simulink model "SIL_Simulation_Parallel_Implementation"  (R2018b)
settings: Solver=FixedStepAuto  StartTime=0.0  StopTime=5  FixedStep=sim_step  RelTol=1e-3
values from neighbouring files (symbols this model uses):
  sim_step = 0.02    [main.m]
settings Model: ExtModeTrigDuration=200  Creator=young  LastModifiedBy=computation
settings DataIOCC: SaveOutput=off  SaveTime=off
settings OptimizationCC: DefaultParameterBehavior=Inlined  UseDivisionForNetSlopeComputation=on  UseFloatMulNetSlope=on  InlineInvariantSignals=on  EnhancedBackFolding=on  BooleansAsBitfields=on  PassReuseOutputArgsAs=Individual arguments  StateBitsets=on  DataBitsets=on  ZeroExternalMemoryAtStartup=off  ZeroInternalMemoryAtStartup=off  NoFixptDivByZeroProtection=on  EfficientFloat2IntCast=on  LifeSpan=1  OptimizeBlockOrder=speed  DifferentSizesBufferReuse=on
settings DebuggingCC: ParameterTunabilityLossMsg=error
settings HardwareCC: ProdBitPerPointer=32  ProdBitPerSizeT=32  ProdBitPerPtrDiffT=32  ProdLargestAtomicInteger=Integer  ProdWordSize=32  ProdLongLongMode=on  ProdHWDeviceType=Custom Processor
settings SFSimCC: SimUseLocalCustomCode=off  MATLABDynamicMemAlloc=off
settings RTWCC: SystemTargetFile=CompSOC_ec.tlc  TemplateMakefile=CompSOC_ec.tmf  Description=CompSOC EC Target  GenerateReport=on  RTWUseLocalCustomCode=off  IncludeHyperlinkInReport=on  LaunchReport=on  CreateSILPILBlock=PIL  CodeExecutionProfiling=on  CodeProfilingSaveOptions=AllData  CodeProfilingInstrumentation=detailed  GenerateTraceInfo=on  GenerateTraceReport=on  GenerateTraceReportSl=on  GenerateTraceReportSf=on  GenerateTraceReportEml=on  GenerateWebview=on  GenerateCodeMetricsReport=on
settings CodeAppCC: ForceParamTrailComments=on  IgnoreCustomStorageClasses=off  OperatorAnnotations=on  SimulinkDataObjDesc=on  SFDataObjDesc=on  CustomSymbolStrGlobalVar=rt$N$M  CustomSymbolStrType=$N$M  CustomSymbolStrFcn=$N$M$F  CustomSymbolStrMacro=$N$M  InsertBlockDesc=on
settings STFCustomTargetCC: TargetLibSuffix=.a  TargetLangStandard=C99 (ISO)  MultiwordLength=256  GenerateSampleERTMain=on  IncludeMdlTerminateFcn=off  CombineOutputUpdateFcns=on  CombineSignalStateStructs=on  ERTCustomFileBanners=on  RemoveResetFunc=on  MATLABClassNameForMDSCustomization=Simulink.SoftwareTarget.ERTCustomization  SystemTargetFile=CompSOC_ec.tlc
settings ERTTargetCC: TargetLangStandard=C99 (ISO)  GenerateSampleERTMain=on  ParMdlRefBuildCompliant=off  CompOptLevelCompliant=off  ConcurrentExecutionCompliant=off  IncludeMdlTerminateFcn=off  CombineSignalStateStructs=on  SupportContinuousTime=on  SupportNonInlinedSFcns=on  ModelStepFunctionPrototypeControlCompliant=off  CPPClassGenCompliant=off  UseToolchainInfoCompliant=off  ExtModeStaticAlloc=on  ExtModeStaticAllocSize=9200  ExtModeMexArgs='pato-board.local' 1 9878  InlinedParameterPlacement=NonHierarchical  ERTCustomFileTemplate=CompSOC_ec_file_process.tlc  ERTFilePackagingFormat=CompactWithDataFile

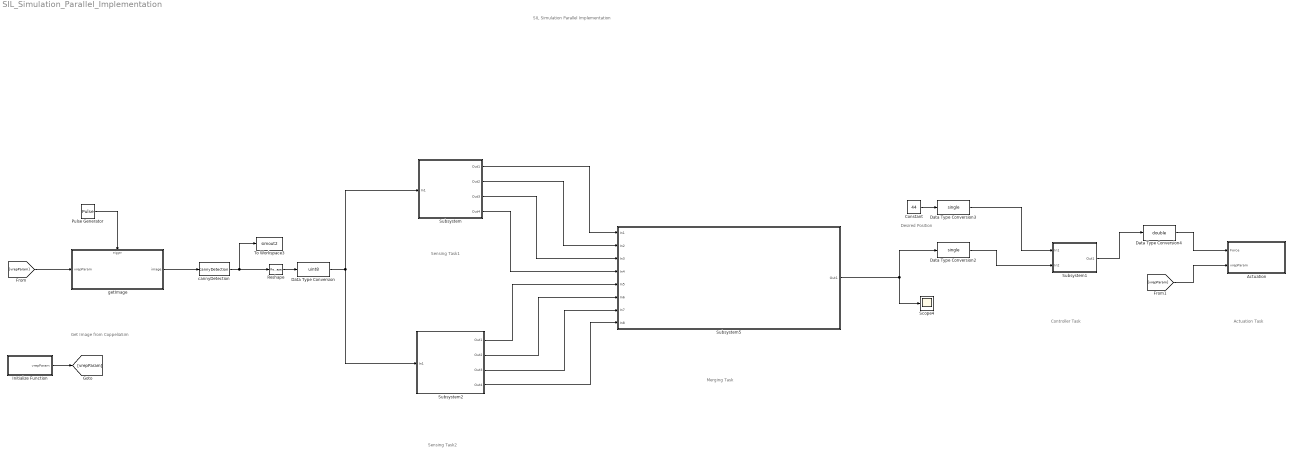
== system SIL_Simulation_Parallel_Implementation ==
  note: SIL Simulation
      | Parallel Implementation
  note: Get Image from CoppeliaSim
  note: Sensing Task1
  note: Sensing Task2
  note: Merging Task
  note: Controller Task
  note: Actuation Task
  note: Desired Position
  Actuation : Subsystem
  Constant : Constant  Value=44
  Data Type Conversion : DataTypeConversion  OutDataTypeStr=uint8
  Data Type Conversion2 : DataTypeConversion  OutDataTypeStr=single
  Data Type Conversion3 : DataTypeConversion  OutDataTypeStr=single
  Data Type Conversion4 : DataTypeConversion  OutDataTypeStr=double
  Initialize Function : Subsystem  TreatAsAtomicUnit=on
  Pulse Generator : DiscretePulseGenerator  SampleTime=sim_step
  Reshape : Reshape
  Scope4 : Scope
  Subsystem : Subsystem
  Subsystem1 : Subsystem
  Subsystem2 : Subsystem
  Subsystem5 : Subsystem
  To Workspace3 : ToWorkspace  VariableName=simout2  SampleTime=-1
      settings: MaxDataPoints=1
  "cannyDetection " : MATLABFcn  MATLABFcn=cannyDetection  OutputDimensions=[142,88]  Output1D=off
  getImage : Subsystem
  wires:
  Reshape/1 -> Data Type Conversion/1
  Initialize Function/1("vrepParam ") -> [vrepParam]
  [vrepParam] -> Actuation/2(vrepParam)
  [vrepParam] -> getImage/1(vrepParam)
  "cannyDetection "/1 -> To Workspace3/1, Reshape/1
  Pulse Generator/1 -> getImage/Trigger
  getImage/1(image) -> "cannyDetection "/1
  Constant/1 -> Data Type Conversion3/1
  Data Type Conversion4/1 -> Actuation/1(Force)
  Data Type Conversion/1 -> Subsystem2/1(In1), Subsystem/1(In1)
  Subsystem5/1(Out1) -> Scope4/1, Data Type Conversion2/1
  Subsystem/1(Out1) -> Subsystem5/1(In1)
  Subsystem/2(Out2) -> Subsystem5/2(In2)
  Subsystem/3(Out3) -> Subsystem5/3(In3)
  Subsystem/4(Out4) -> Subsystem5/4(In4)
  Subsystem2/1(Out1) -> Subsystem5/5(In5)
  Subsystem2/2(Out2) -> Subsystem5/6(In6)
  Subsystem2/3(Out3) -> Subsystem5/7(In7)
  Subsystem2/4(Out4) -> Subsystem5/8(In8)
  Data Type Conversion3/1 -> Subsystem1/1(In1)
  Data Type Conversion2/1 -> Subsystem1/2(In2)
  Subsystem1/1(Out1) -> Data Type Conversion4/1

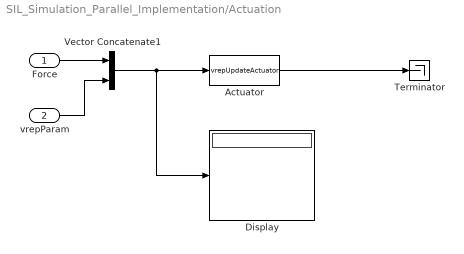
== system SIL_Simulation_Parallel_Implementation/Actuation ==
  Force : Inport
  vrepParam : Inport  Port=2
  "Actuator " : MATLABFcn  MATLABFcn=vrepUpdateActuator  OutputDimensions=1  Output1D=off
  Display : Display
  Terminator : Terminator
  Vector Concatenate1 : Concatenate
  wires:
  vrepParam/1 -> Vector Concatenate1/2
  Force/1 -> Vector Concatenate1/1
  Vector Concatenate1/1 -> Display/1, "Actuator "/1
  "Actuator "/1 -> Terminator/1

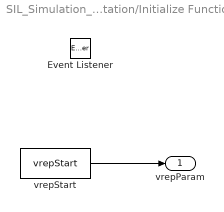
== system SIL_Simulation_Parallel_Implementation/Initialize Function ==
  Event Listener : EventListener  DisableCoverage=on  EventName=reset
  "vrepStart " : MATLABFcn  MATLABFcn=vrepStart
  "vrepParam " : Outport
  wires:
  "vrepStart "/1 -> "vrepParam "/1

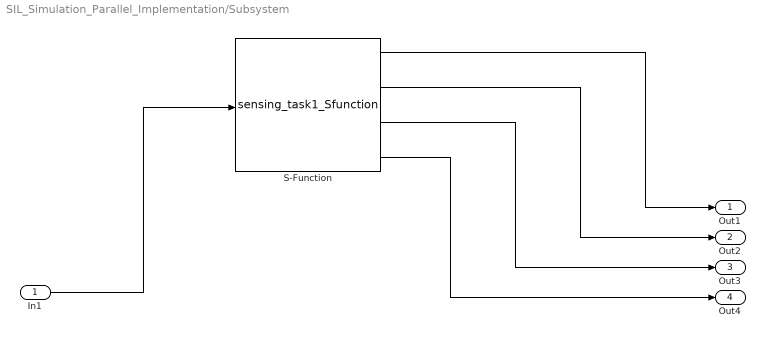
== system SIL_Simulation_Parallel_Implementation/Subsystem ==
  In1 : Inport
  S-Function : S-Function  FunctionName=sensing_task1_Sfunction  SFunctionDeploymentMode=off  EnableBusSupport=off
  Out1 : Outport
  Out2 : Outport  Port=2
  Out3 : Outport  Port=3
  Out4 : Outport  Port=4
  wires:
  S-Function/4 -> Out4/1
  In1/1 -> S-Function/1
  S-Function/1 -> Out1/1
  S-Function/3 -> Out3/1
  S-Function/2 -> Out2/1

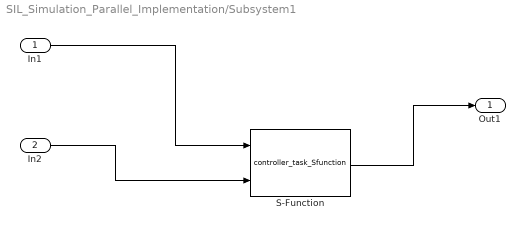
== system SIL_Simulation_Parallel_Implementation/Subsystem1 ==
  In1 : Inport
  In2 : Inport  Port=2
  S-Function : S-Function  FunctionName=controller_task_Sfunction  SFunctionDeploymentMode=off  EnableBusSupport=off
  Out1 : Outport
  wires:
  S-Function/1 -> Out1/1
  In2/1 -> S-Function/2
  In1/1 -> S-Function/1

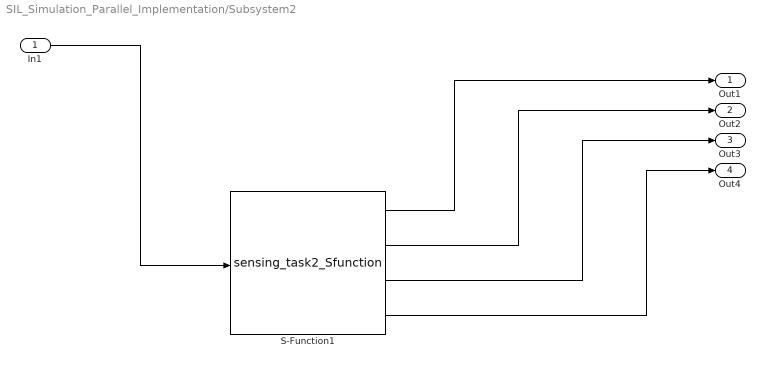
== system SIL_Simulation_Parallel_Implementation/Subsystem2 ==
  In1 : Inport
  S-Function1 : S-Function  FunctionName=sensing_task2_Sfunction  SFunctionDeploymentMode=off  EnableBusSupport=off
  Out1 : Outport
  Out2 : Outport  Port=2
  Out3 : Outport  Port=3
  Out4 : Outport  Port=4
  wires:
  S-Function1/4 -> Out4/1
  S-Function1/2 -> Out2/1
  S-Function1/3 -> Out3/1
  In1/1 -> S-Function1/1
  S-Function1/1 -> Out1/1

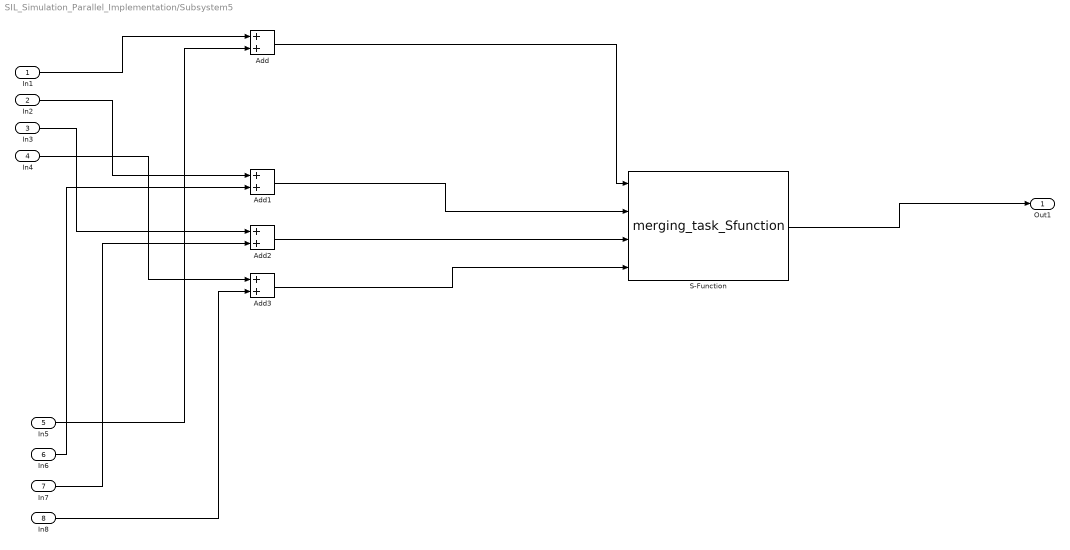
== system SIL_Simulation_Parallel_Implementation/Subsystem5 ==
  In1 : Inport
  In2 : Inport  Port=2
  In3 : Inport  Port=3
  In4 : Inport  Port=4
  In5 : Inport  Port=5
  In6 : Inport  Port=6
  In7 : Inport  Port=7
  In8 : Inport  Port=8
  Add{,1..3} (4 alike) : Sum
  S-Function : S-Function  FunctionName=merging_task_Sfunction  SFunctionDeploymentMode=off  EnableBusSupport=off
  Out1 : Outport
  wires:
  In8/1 -> Add3/2
  In4/1 -> Add3/1
  In2/1 -> Add1/1
  Add2/1 -> S-Function/3
  In6/1 -> Add1/2
  In7/1 -> Add2/2
  In5/1 -> Add/2
  Add3/1 -> S-Function/4
  S-Function/1 -> Out1/1
  Add/1 -> S-Function/1
  In3/1 -> Add2/1
  Add1/1 -> S-Function/2
  In1/1 -> Add/1

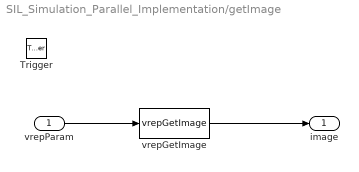
== system SIL_Simulation_Parallel_Implementation/getImage ==
  vrepParam : Inport
  Trigger : TriggerPort  VariantControl=Variant  PortDimensions=1
  vrepGetImage : MATLABFcn  MATLABFcn=vrepGetImage  OutputDimensions=[142,88]  Output1D=off
  image : Outport
  wires:
  vrepParam/1 -> vrepGetImage/1
  vrepGetImage/1 -> image/1
